simulink model "sl_R3GDL_MFunction"  (Simulink 8.9)
settings: Solver=ode45  StartTime=0.0  StopTime=tsim  RelTol=1e-8  EnableMultiTasking=on
settings Model: Creator=Manuel G. Ortega  LastModifiedBy=Javi Gómez  ExtModeTrigMode=oneshot  ExtModeArmWhenConnect=off
settings DataIOCC: LimitDataPoints=off
settings OptimizationCC: BooleanDataType=off  ExpressionDepthLimit=2147483647  InitFltsAndDblsToZero=on
settings DebuggingCC: SaveWithParameterizedLinksMsg=none  SignalResolutionControl=TryResolveAllWithWarning  MultiTaskDSMMsg=warning  MultiTaskCondExecSysMsg=none
settings HardwareCC: TargetUnknown=on
settings GRTTargetCC: TargetFcnLib=ansi_tfl_tmw.mat
settings ConfigComp: CovSFcnEnable=off

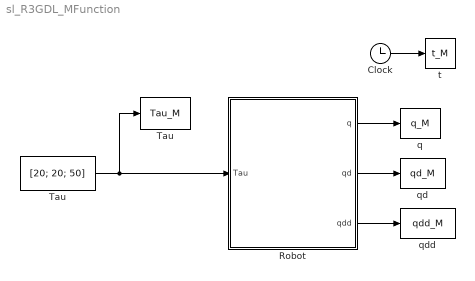
== system sl_R3GDL_MFunction ==
  Clock : Clock
  Robot : Subsystem
  Tau : Constant  Value=[20; 20; 50]  SampleTime=0
  "Tau " : ToWorkspace  VariableName=Tau_M  SampleTime=-1
  q : ToWorkspace  VariableName=q_M  SampleTime=-1
  qd : ToWorkspace  VariableName=qd_M  SampleTime=-1
  qdd : ToWorkspace  VariableName=qdd_M  SampleTime=-1
  t : ToWorkspace  VariableName=t_M  SampleTime=-1
  wires:
  Robot/1(q) -> q/1
  Robot/2(qd) -> qd/1
  Robot/3(qdd) -> qdd/1
  Clock/1 -> t/1
  Tau/1 -> Robot/1(Tau), "Tau "/1

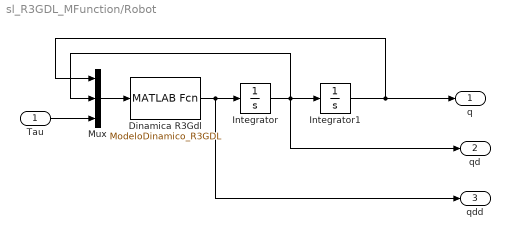
== system sl_R3GDL_MFunction/Robot ==
  Tau : Inport
  Dinamica R3Gdl : MATLABFcn  MATLABFcn=ModeloDinamico_R3GDL
  Integrator : Integrator  InitialCondition=[0;0;0];
  Integrator1 : Integrator  InitialCondition=[0;0;0]
  Mux : Mux  Inputs=3
  q : Outport
  qd : Outport  Port=2
  qdd : Outport  Port=3
  wires:
  Mux/1 -> Dinamica R3Gdl/1
  Dinamica R3Gdl/1 -> Integrator/1, qdd/1
  Integrator/1 -> Integrator1/1, qd/1, Mux/2
  Integrator1/1 -> q/1, Mux/1
  Tau/1 -> Mux/3
